simulink model "PendulumFriction"  (Simulink 8.6)
settings: Solver=ode1  SolverMode=SingleTasking  StartTime=0.0  StopTime=25  FixedStep=0.001  RelTol=1e-3
undefined symbols (not defined in the file): Advantech, PCI
libraries: sldrtlib x11, simulink x8
settings Model: Creator=Demo11  LastModifiedBy=demo  SimulationMode=external  ExtModeTrigMode=oneshot  ExtModeTrigDuration=100000
settings DataIOCC: LimitDataPoints=off  SignalLoggingName=sigsOut
settings OptimizationCC: BlockReduction=off  BooleanDataType=off  InitFltsAndDblsToZero=on
settings DebuggingCC: SaveWithParameterizedLinksMsg=none  SignalResolutionControl=TryResolveAllWithWarning  SolverPrmCheckMsg=none  MultiTaskDSMMsg=warning  MultiTaskCondExecSysMsg=none  FcnCallInpInsideContextMsg=UseLocalSettings
settings HardwareCC: ProdBitPerLong=64  ProdBitPerPointer=64  ProdIntDivRoundTo=Zero  ProdEndianess=LittleEndian  ProdWordSize=64  ProdHWDeviceType=Intel->x86-64  TargetBitPerLong=64  TargetBitPerPointer=64  TargetIntDivRoundTo=Zero  TargetEndianess=LittleEndian  TargetWordSize=64  TargetHWDeviceType=Intel->x86-64
settings RTWCC: SystemTargetFile=sldrt.tlc  TemplateMakefile=sldrt.tmf  Description=Simulink Desktop Real-Time  RTWCompilerOptimization=on
settings CodeAppCC: MaxIdLength=95
settings SimulinkDesktopRealTimeCC: TargetPreCompLibLocation=C:\Program Files\MATLAB\R2015b\toolbox\sldrt\lib\win64  TargetLangStandard=C89/C90 (ANSI)  SupportVariableSizeSignals=off

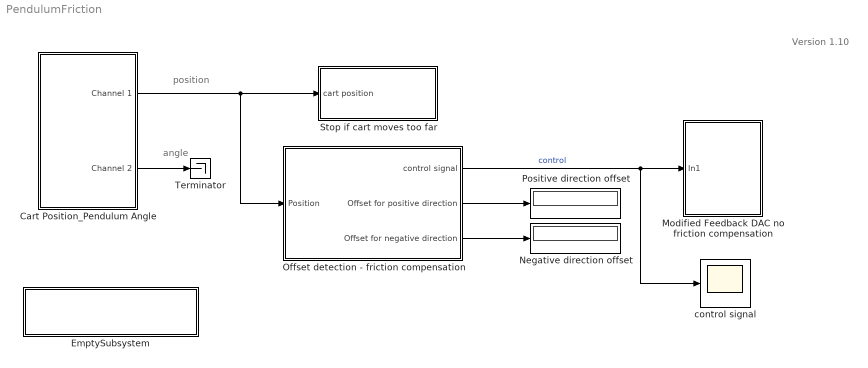
== system PendulumFriction ==
  note: position
  note: angle
  note: Version 1.10
  Cart Position_Pendulum Angle : Subsystem  mask(Feedback Encoder Block){st=0.001, of1=0, of2=-1024}
      mask prompts: st "Sample Time"; of1 "Channel 1 Offset"; of2 "Channel 2 Offset"
      mask help: Special block to use with the Feedback experiments to read encoder channels using the digital I/O lines
      mask Display:
      | image(imread('bckg.bmp'))
      | disp('PCI1711 \n Lab I/O Board \n\n\n Feedback Encoder')
  EmptySubsystem : Subsystem
      mask Display:
      | image(imread('FB-inst-blue2.jpg'))
      | disp('\n\nFeedback Instruments Limited')
  Modified Feedback DAC no friction compensation : Subsystem  mask(DAC Unit for Feedback Experiments){st=0.001, ch=1}
      mask prompts: st "Sample Time"; ch "Output Channel"
      mask help:
      | Digital to Analog Output  for Feedback Experiments
      | using Advantech PCI1711  I/O board
      mask Display: disp('PCI1711 \n Lab I/O Board \n\n Feedback  DAC')
  Negative direction offset : Display
      settings: SampleTime=0.01
  Offset detection - friction compensation : Subsystem
      mask Display:
      | image(imread('bckg.bmp'))
      | disp('Offset detection')
  Positive direction offset : Display
      settings: SampleTime=0.01
  Stop if cart moves too far : Subsystem
      mask Display:
      | image(imread('bckg.bmp'))
      | disp('Safety stop')
  Terminator : Terminator
  control signal : Scope
      mask Display: image(imread('scope.jpg'))
  wires:
  Cart Position_Pendulum Angle/1(Channel 1) -> Stop if cart moves too far/1(cart position), Offset detection - friction compensation/1(Position)
  Cart Position_Pendulum Angle/2(Channel 2) -> Terminator/1
  Offset detection - friction compensation/2(Offset for positive direction) -> Positive direction offset/1
  Offset detection - friction compensation/3(Offset for negative direction) -> Negative direction offset/1
  Offset detection - friction compensation/1(control signal) -> control signal/1, Modified Feedback DAC no friction compensation/1(In1)  "control"

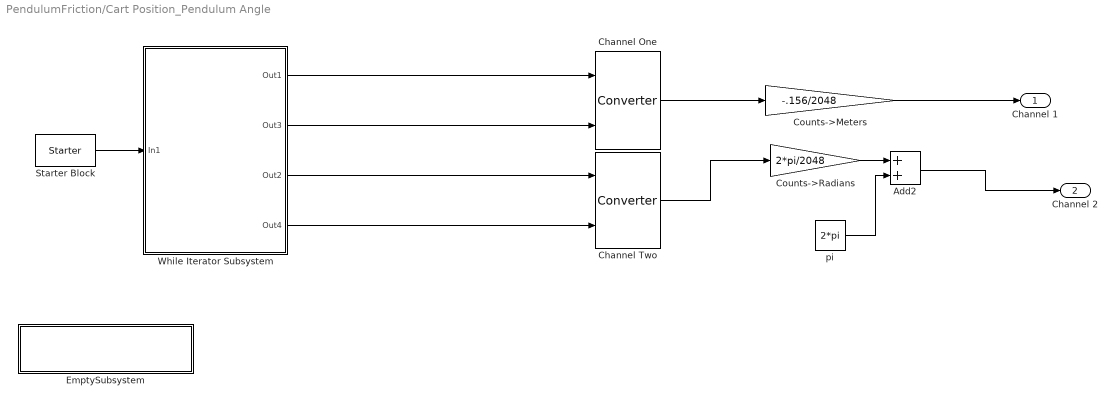
== system PendulumFriction/Cart Position_Pendulum Angle ==
  Add2 : Sum
  Channel One : S-Function  FunctionName=Converter  Parameters=of1,st  SFunctionDeploymentMode=off  EnableBusSupport=off
  Channel Two : S-Function  FunctionName=Converter  Parameters=of2,st  SFunctionDeploymentMode=off  EnableBusSupport=off
  Counts->Meters : Gain  Gain=-.156/2048  SaturateOnIntegerOverflow=on  OutDataTypeStr=Inherit: Same as input  ParamDataTypeStr=Inherit: Same as input
  Counts->Radians : Gain  Gain=2*pi/2048  SaturateOnIntegerOverflow=on  OutDataTypeStr=Inherit: Same as input  ParamDataTypeStr=Inherit: Same as input
  EmptySubsystem : Subsystem
      mask Display:
      | image(imread('FB-inst-blue2.jpg'))
      | disp('\n\nFeedback Instruments Limited')
  Starter Block : S-Function  FunctionName=Starter  Parameters=sample_time  SFunctionDeploymentMode=off  EnableBusSupport=off  mask{sample_time=st}
      mask prompts: sample_time "Sample Time:"
  While Iterator Subsystem : Subsystem  TreatAsAtomicUnit=on
  pi : Constant  Value=2*pi
  Channel 1 : Outport
  Channel 2 : Outport  Port=2
  wires:
  Add2/1 -> Channel 2/1
  Channel Two/1 -> Counts->Radians/1
  pi/1 -> Add2/2
  Counts->Radians/1 -> Add2/1
  Counts->Meters/1 -> Channel 1/1
  Starter Block/1 -> While Iterator Subsystem/1(In1)
  While Iterator Subsystem/1(Out1) -> Channel One/1
  While Iterator Subsystem/2(Out3) -> Channel One/2
  While Iterator Subsystem/3(Out2) -> Channel Two/1
  While Iterator Subsystem/4(Out4) -> Channel Two/2
  Channel One/1 -> Counts->Meters/1

== system PendulumFriction/EmptySubsystem ==

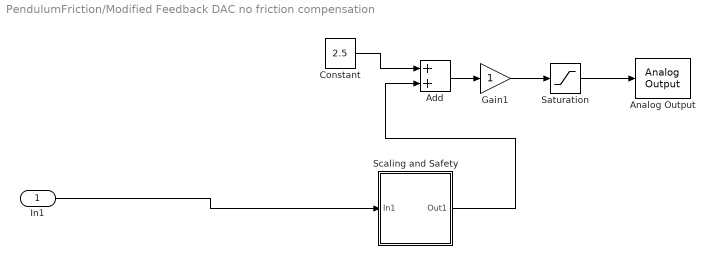
== system PendulumFriction/Modified Feedback DAC no friction compensation ==
  In1 : Inport
  Add : Sum  OutDataTypeStr=Inherit: Same as first input
  Analog Output : sldrtlib/Analog Output  SampleTime=st  MaxMissedTicks=10  ShowMissedTicks=off  YieldWhenWaiting=off  DrvName=Advantech/PCI-1711  DrvAddress=4294967295  DrvOptions=zeros(1,0)  Channels=ch  RangeMode=1  VoltRange=2  InitialValue=2.5  FinalValue=2.5
      settings: AttributesFormatString=Advantech\nPCI-1711 [auto]
  Constant : Constant  Value=2.5
  Gain1 : Gain
  Saturation : Saturate  UpperLimit=5.0  LowerLimit=0
  Scaling and Safety : Subsystem
  wires:
  Constant/1 -> Add/1
  Saturation/1 -> Analog Output/1
  Add/1 -> Gain1/1
  Gain1/1 -> Saturation/1
  Scaling and Safety/1(Out1) -> Add/2
  In1/1 -> Scaling and Safety/1(In1)

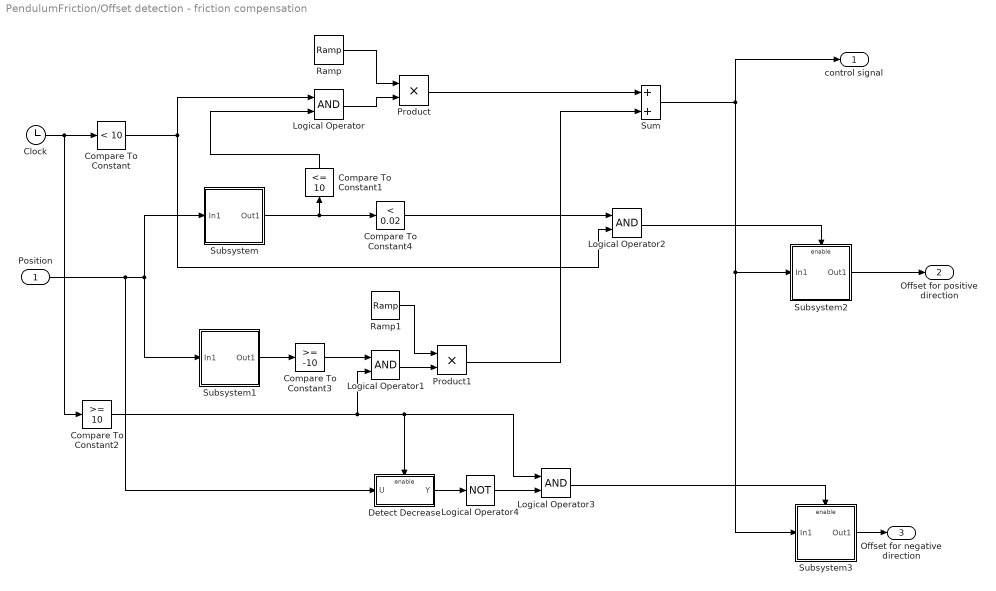
== system PendulumFriction/Offset detection - friction compensation ==
  Position : Inport
  Clock : Clock
  Compare To Constant : simulink/Logic and Bit Operations/Compare To Constant  relop=<  const=10  OutDataTypeStr=boolean  ZeroCross=off
  Compare To Constant1 : simulink/Logic and Bit Operations/Compare To Constant  relop=<=  const=10  OutDataTypeStr=boolean  ZeroCross=off
  Compare To Constant2 : simulink/Logic and Bit Operations/Compare To Constant  relop=>=  const=10  OutDataTypeStr=boolean  ZeroCross=off
  Compare To Constant3 : simulink/Logic and Bit Operations/Compare To Constant  relop=>=  const=-10  OutDataTypeStr=boolean  ZeroCross=off
  Compare To Constant4 : simulink/Logic and Bit Operations/Compare To Constant  relop=<  const=0.02  OutDataTypeStr=boolean  ZeroCross=off
  Detect Decrease : Subsystem  AncestorBlock=|  TreatAsAtomicUnit=on  mask(Detect Decrease){vinit=0.0}
      | simulink/Logic and Bit
      | Operations/Detect
      | Decrease
      mask prompts: vinit "Initial condition:"
      mask help: If the input is strictly less than its previous value, then output TRUE, otherwise output FALSE. The initial condition determines the initial value of the previous input U/z.
      mask Display: fprintf('U < U/z')
  Logical Operator{,1..3} (4 alike) : Logic  AllPortsSameDT=off  OutDataTypeStr=boolean
  Logical Operator4 : Logic  Operator=NOT  AllPortsSameDT=off  OutDataTypeStr=boolean
  Product : Product  RndMeth=Zero
  Product1 : Product  RndMeth=Zero
  Ramp : simulink/Sources/Ramp  slope=0.02  start=0  X0=0
  Ramp1 : simulink/Sources/Ramp  slope=-0.02  start=10  X0=0
  Subsystem : Subsystem  TreatAsAtomicUnit=on
  Subsystem1 : Subsystem  TreatAsAtomicUnit=on
  Subsystem2 : Subsystem  TreatAsAtomicUnit=on
  Subsystem3 : Subsystem  TreatAsAtomicUnit=on
  Sum : Sum
  control signal : Outport
  Offset for positive direction : Outport  Port=2
  Offset for negative direction : Outport  Port=3
  wires:
  Clock/1 -> Compare To Constant/1, Compare To Constant2/1
  Ramp/1 -> Product/1
  Compare To Constant1/1 -> Logical Operator/2
  Compare To Constant/1 -> Logical Operator2/2, Logical Operator/1
  Logical Operator/1 -> Product/2
  Product/1 -> Sum/1
  Compare To Constant3/1 -> Logical Operator1/1
  Compare To Constant2/1 -> Logical Operator1/2, Detect Decrease/Enable, Logical Operator3/1
  Logical Operator1/1 -> Product1/2
  Ramp1/1 -> Product1/1
  Product1/1 -> Sum/2
  Sum/1 -> Subsystem2/1(In1), Subsystem3/1(In1), control signal/1
  Subsystem1/1(Out1) -> Compare To Constant3/1
  Compare To Constant4/1 -> Logical Operator2/1
  Detect Decrease/1(Y) -> Logical Operator4/1
  Logical Operator3/1 -> Subsystem3/Enable
  Logical Operator4/1 -> Logical Operator3/2
  Position/1 -> Subsystem/1(In1), Subsystem1/1(In1), Detect Decrease/1(U)
  Subsystem2/1(Out1) -> Offset for positive direction/1
  Subsystem3/1(Out1) -> Offset for negative direction/1
  Logical Operator2/1 -> Subsystem2/Enable
  Subsystem/1(Out1) -> Compare To Constant1/1, Compare To Constant4/1

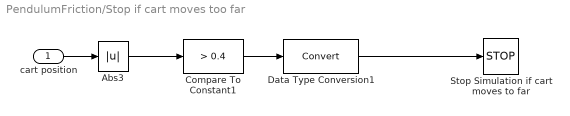
== system PendulumFriction/Stop if cart moves too far ==
  cart position : Inport
  Abs3 : Abs
  Compare To Constant1 : simulink/Logic and Bit Operations/Compare To Constant  relop=>  const=0.4  OutDataTypeStr=boolean  ZeroCross=off
  Data Type Conversion1 : DataTypeConversion
  Stop Simulation if cart moves to far : Stop
  wires:
  Abs3/1 -> Compare To Constant1/1
  Compare To Constant1/1 -> Data Type Conversion1/1
  Data Type Conversion1/1 -> Stop Simulation if cart moves to far/1
  cart position/1 -> Abs3/1

== system PendulumFriction/Cart Position_Pendulum Angle/EmptySubsystem ==

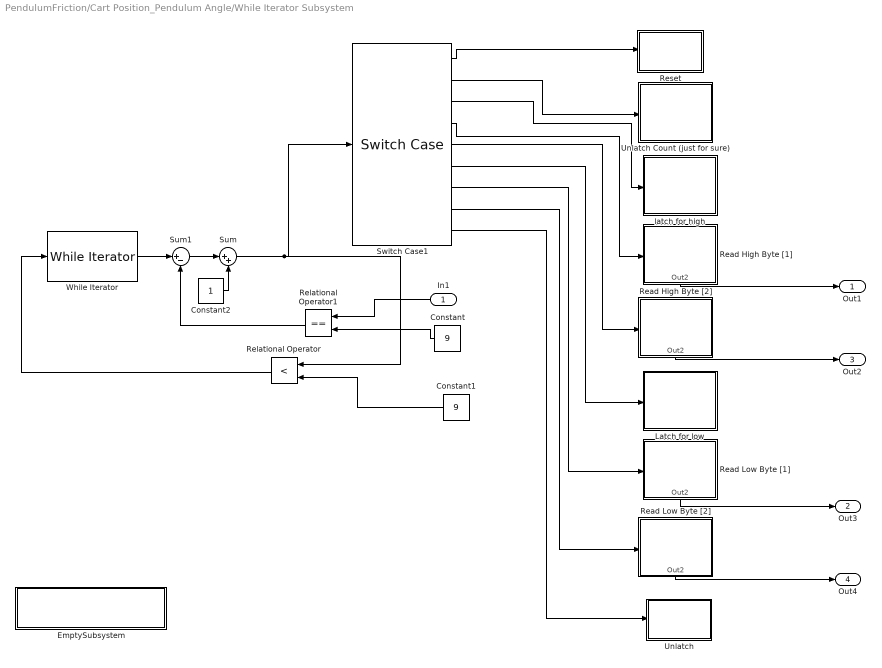
== system PendulumFriction/Cart Position_Pendulum Angle/While Iterator Subsystem ==
  In1 : Inport
  Constant : Constant  Value=9
  Constant1 : Constant  Value=9
  Constant2 : Constant
  EmptySubsystem : Subsystem
      mask Display:
      | image(imread('FB-inst-blue2.jpg'))
      | disp('\n\nFeedback Instruments Limited')
  Latch for low : Subsystem  TreatAsAtomicUnit=on
  Read High Byte [1] : Subsystem  TreatAsAtomicUnit=on
  Read High Byte [2] : Subsystem  TreatAsAtomicUnit=on
  Read Low Byte [1] : Subsystem  TreatAsAtomicUnit=on
  Read Low Byte [2] : Subsystem  TreatAsAtomicUnit=on
  Relational Operator : RelationalOperator  Operator=<  OutDataTypeStr=boolean
  Relational Operator1 : RelationalOperator  Operator===  OutDataTypeStr=boolean
  Reset : Subsystem  TreatAsAtomicUnit=on
  Sum : Sum  Inputs=|++
  Sum1 : Sum  Inputs=|+-  OutDataTypeStr=Inherit: Same as first input
  Switch Case1 : SwitchCase  CaseConditions={1,2,3,4,5,6,7,8,9}  ShowDefaultCase=off
  Unlatch : Subsystem  TreatAsAtomicUnit=on
  "Unlatch Count (just for sure) " : Subsystem  TreatAsAtomicUnit=on
  While Iterator : WhileIterator  MaxIters=9  WhileBlockType=do-while  ResetStates=reset  ShowIterationPort=on  OutputDataType=int8
  latch for high : Subsystem  TreatAsAtomicUnit=on
  Out1 : Outport
  Out3 : Outport  Port=2
  Out2 : Outport  Port=3
  Out4 : Outport  Port=4
  wires:
  Relational Operator/1 -> While Iterator/1
  In1/1 -> Relational Operator1/1
  Constant/1 -> Relational Operator1/2
  Relational Operator1/1 -> Sum1/2
  While Iterator/1 -> Sum1/1
  Switch Case1/1 -> Reset/Action
  Switch Case1/2 -> "Unlatch Count (just for sure) "/Action
  Constant1/1 -> Relational Operator/2
  Read High Byte [1]/1(Out2) -> Out1/1
  Read High Byte [2]/1(Out2) -> Out2/1
  Read Low Byte [1]/1(Out2) -> Out3/1
  Read Low Byte [2]/1(Out2) -> Out4/1
  Sum1/1 -> Sum/1
  Sum/1 -> Switch Case1/1, Relational Operator/1
  Constant2/1 -> Sum/2
  Switch Case1/3 -> latch for high/Action
  Switch Case1/4 -> Read High Byte [1]/Action
  Switch Case1/5 -> Read High Byte [2]/Action
  Switch Case1/6 -> Latch for low/Action
  Switch Case1/7 -> Read Low Byte [1]/Action
  Switch Case1/8 -> Read Low Byte [2]/Action
  Switch Case1/9 -> Unlatch/Action

== system PendulumFriction/Modified Feedback DAC no friction compensation/Scaling and Safety ==
  In1 : Inport
  -1 : Gain  Gain=-1  SaturateOnIntegerOverflow=on  OutDataTypeStr=Inherit: Same as input  ParamDataTypeStr=Inherit: Same as input
  Saturation : Saturate  UpperLimit=2.5  LowerLimit=-2.5
  Out1 : Outport
  wires:
  -1/1 -> Saturation/1  "actual LoadPosition"
  In1/1 -> -1/1
  Saturation/1 -> Out1/1

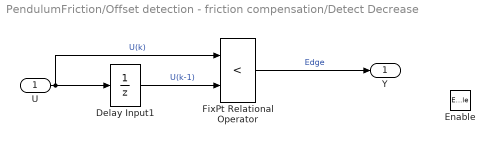
== system PendulumFriction/Offset detection - friction compensation/Detect Decrease ==
  U : Inport
  Enable : EnablePort
  Delay Input1 : UnitDelay  Description=Store in Global RAM  InitialCondition=vinit  SampleTime=-1
  FixPt Relational Operator : RelationalOperator  Operator=<  OutDataTypeStr=uint(8)  ZeroCross=off
  Y : Outport  InitialOutput=0
  wires:
  U/1 -> Delay Input1/1, FixPt Relational Operator/1  "U(k)"
  Delay Input1/1 -> FixPt Relational Operator/2  "U(k-1)"
  FixPt Relational Operator/1 -> Y/1  "Edge"

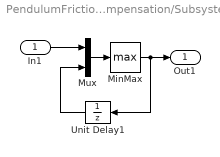
== system PendulumFriction/Offset detection - friction compensation/Subsystem ==
  In1 : Inport
  MinMax : MinMax  Function=max
  Mux : Mux  Inputs=2
  Unit Delay1 : UnitDelay  SampleTime=0.01
  Out1 : Outport
  wires:
  In1/1 -> Mux/1
  Unit Delay1/1 -> Mux/2
  Mux/1 -> MinMax/1
  MinMax/1 -> Out1/1, Unit Delay1/1

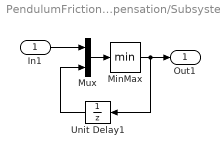
== system PendulumFriction/Offset detection - friction compensation/Subsystem1 ==
  In1 : Inport
  MinMax : MinMax
  Mux : Mux  Inputs=2
  Unit Delay1 : UnitDelay  SampleTime=0.01
  Out1 : Outport
  wires:
  MinMax/1 -> Unit Delay1/1, Out1/1
  Mux/1 -> MinMax/1
  Unit Delay1/1 -> Mux/2
  In1/1 -> Mux/1

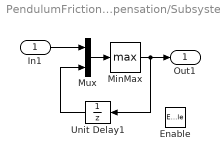
== system PendulumFriction/Offset detection - friction compensation/Subsystem2 ==
  In1 : Inport
  Enable : EnablePort
  MinMax : MinMax  Function=max
  Mux : Mux  Inputs=2
  Unit Delay1 : UnitDelay  SampleTime=0.01
  Out1 : Outport
  wires:
  In1/1 -> Mux/1
  Unit Delay1/1 -> Mux/2
  Mux/1 -> MinMax/1
  MinMax/1 -> Out1/1, Unit Delay1/1

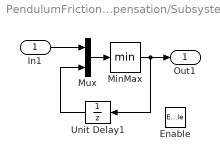
== system PendulumFriction/Offset detection - friction compensation/Subsystem3 ==
  In1 : Inport
  Enable : EnablePort
  MinMax : MinMax
  Mux : Mux  Inputs=2
  Unit Delay1 : UnitDelay  SampleTime=0.01
  Out1 : Outport
  wires:
  MinMax/1 -> Unit Delay1/1, Out1/1
  Mux/1 -> MinMax/1
  Unit Delay1/1 -> Mux/2
  In1/1 -> Mux/1

== system PendulumFriction/Cart Position_Pendulum Angle/While Iterator Subsystem/EmptySubsystem ==

== system PendulumFriction/Cart Position_Pendulum Angle/While Iterator Subsystem/Latch for low ==
  Action Port : ActionPort  ActionType=case
  Constant : Constant  Value=6  OutDataTypeStr=double
  Digital Output : sldrtlib/Digital Output  SampleTime=-1  MaxMissedTicks=10  ShowMissedTicks=off  YieldWhenWaiting=off  DrvName=Advantech/PCI-1711  DrvAddress=4294967295  DrvOptions=zeros(1,0)  Channels=1  BitMode=2  InitialValue=0  FinalValue=0
      settings: AttributesFormatString=Advantech\nPCI-1711 [auto]
  wires:
  Constant/1 -> Digital Output/1

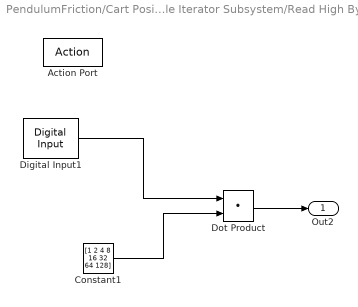
== system PendulumFriction/Cart Position_Pendulum Angle/While Iterator Subsystem/Read High Byte [1] ==
  Action Port : ActionPort  ActionType=case
  Constant1 : Constant  Value=[1 2 4 8 16 32 64 128]
  Digital Input1 : sldrtlib/Digital Input  SampleTime=-1  MaxMissedTicks=10  ShowMissedTicks=off  YieldWhenWaiting=off  DrvName=Advantech/PCI-1711  DrvAddress=4294967295  DrvOptions=zeros(1,0)  Channels=[1,2,3,4,5,6,7,8]  BitMode=1  DataType=1
      settings: AttributesFormatString=Advantech\nPCI-1711 [auto]
  Dot Product : DotProduct  InputSameDT=on  OutDataTypeStr=Inherit: Inherit via internal rule
  Out2 : Outport
  wires:
  Dot Product/1 -> Out2/1
  Constant1/1 -> Dot Product/2
  Digital Input1/1 -> Dot Product/1

== system PendulumFriction/Cart Position_Pendulum Angle/While Iterator Subsystem/Read High Byte [2] ==
  Action Port : ActionPort  ActionType=case
  Constant1 : Constant  Value=[1 2 4 8 16 32 64 128]
  Digital Input1 : sldrtlib/Digital Input  SampleTime=-1  MaxMissedTicks=10  ShowMissedTicks=off  YieldWhenWaiting=off  DrvName=Advantech/PCI-1711  DrvAddress=4294967295  DrvOptions=zeros(1,0)  Channels=[9:16]  BitMode=1  DataType=1
      settings: AttributesFormatString=Advantech\nPCI-1711 [auto]
  Dot Product : DotProduct  InputSameDT=on  OutDataTypeStr=Inherit: Inherit via internal rule
  Out2 : Outport
  wires:
  Digital Input1/1 -> Dot Product/1
  Constant1/1 -> Dot Product/2
  Dot Product/1 -> Out2/1

== system PendulumFriction/Cart Position_Pendulum Angle/While Iterator Subsystem/Read Low Byte [1] ==
  Action Port : ActionPort  ActionType=case
  Constant1 : Constant  Value=[1 2 4 8 16 32 64 128]
  Digital Input1 : sldrtlib/Digital Input  SampleTime=-1  MaxMissedTicks=10  ShowMissedTicks=off  YieldWhenWaiting=off  DrvName=Advantech/PCI-1711  DrvAddress=4294967295  DrvOptions=zeros(1,0)  Channels=[1:8]  BitMode=1  DataType=1
      settings: AttributesFormatString=Advantech\nPCI-1711 [auto]
  Dot Product : DotProduct  InputSameDT=on  OutDataTypeStr=Inherit: Inherit via internal rule
  Out2 : Outport
  wires:
  Digital Input1/1 -> Dot Product/1
  Constant1/1 -> Dot Product/2
  Dot Product/1 -> Out2/1

== system PendulumFriction/Cart Position_Pendulum Angle/While Iterator Subsystem/Read Low Byte [2] ==
  Action Port : ActionPort  ActionType=case
  Constant1 : Constant  Value=[1 2 4 8 16 32 64 128]
  Digital Input1 : sldrtlib/Digital Input  SampleTime=-1  MaxMissedTicks=10  ShowMissedTicks=off  YieldWhenWaiting=off  DrvName=Advantech/PCI-1711  DrvAddress=4294967295  DrvOptions=zeros(1,0)  Channels=[9:16]  BitMode=1  DataType=1
      settings: AttributesFormatString=Advantech\nPCI-1711 [auto]
  Dot Product : DotProduct  InputSameDT=on  OutDataTypeStr=Inherit: Inherit via internal rule
  Out2 : Outport
  wires:
  Constant1/1 -> Dot Product/2
  Digital Input1/1 -> Dot Product/1
  Dot Product/1 -> Out2/1

== system PendulumFriction/Cart Position_Pendulum Angle/While Iterator Subsystem/Reset ==
  Action Port : ActionPort  ActionType=case
  Constant : Constant  Value=3  OutDataTypeStr=double
  Digital Output1 : sldrtlib/Digital Output  SampleTime=-1  MaxMissedTicks=10  ShowMissedTicks=off  YieldWhenWaiting=off  DrvName=Advantech/PCI-1711  DrvAddress=4294967295  DrvOptions=zeros(1,0)  Channels=1  BitMode=2  InitialValue=0  FinalValue=0
      settings: AttributesFormatString=Advantech\nPCI-1711 [auto]
  Subsystem : Subsystem
  wires:
  Constant/1 -> Subsystem/1(In1)
  Subsystem/1(Out1) -> Digital Output1/1

== system PendulumFriction/Cart Position_Pendulum Angle/While Iterator Subsystem/Unlatch ==
  Action Port : ActionPort  ActionType=case
  Constant : Constant  Value=7  OutDataTypeStr=double
  Digital Output1 : sldrtlib/Digital Output  SampleTime=-1  MaxMissedTicks=10  ShowMissedTicks=off  YieldWhenWaiting=off  DrvName=Advantech/PCI-1711  DrvAddress=4294967295  DrvOptions=zeros(1,0)  Channels=1  BitMode=2  InitialValue=0  FinalValue=0
      settings: AttributesFormatString=Advantech\nPCI-1711 [auto]
  wires:
  Constant/1 -> Digital Output1/1

== system PendulumFriction/Cart Position_Pendulum Angle/While Iterator Subsystem/Unlatch Count (just for sure)  ==
  Action Port : ActionPort  ActionType=case
  Constant : Constant  Value=7  OutDataTypeStr=double
  Digital Output : sldrtlib/Digital Output  SampleTime=-1  MaxMissedTicks=10  ShowMissedTicks=off  YieldWhenWaiting=off  DrvName=Advantech/PCI-1711  DrvAddress=4294967295  DrvOptions=zeros(1,0)  Channels=1  BitMode=2  InitialValue=0  FinalValue=0
      settings: AttributesFormatString=Advantech\nPCI-1711 [auto]
  wires:
  Constant/1 -> Digital Output/1

== system PendulumFriction/Cart Position_Pendulum Angle/While Iterator Subsystem/latch for high ==
  Action Port : ActionPort  ActionType=case
  Constant : Constant  Value=4  OutDataTypeStr=double
  Digital Output : sldrtlib/Digital Output  SampleTime=-1  MaxMissedTicks=10  ShowMissedTicks=off  YieldWhenWaiting=off  DrvName=Advantech/PCI-1711  DrvAddress=4294967295  DrvOptions=zeros(1,0)  Channels=1  BitMode=2  InitialValue=0  FinalValue=0
      settings: AttributesFormatString=Advantech\nPCI-1711 [auto]
  wires:
  Constant/1 -> Digital Output/1

== system PendulumFriction/Cart Position_Pendulum Angle/While Iterator Subsystem/Reset/Subsystem ==
  In1 : Inport
  Constant1 : Constant  Value=7  OutDataTypeStr=double
  Digital Output : sldrtlib/Digital Output  SampleTime=-1  MaxMissedTicks=10  ShowMissedTicks=off  YieldWhenWaiting=off  DrvName=Advantech/PCI-1711  DrvAddress=4294967295  DrvOptions=zeros(1,0)  Channels=[1 2 3]  BitMode=2  InitialValue=0  FinalValue=0
      settings: AttributesFormatString=Advantech\nPCI-1711 [auto]
  Out1 : Outport
  wires:
  Constant1/1 -> Out1/1
  In1/1 -> Digital Output/1
